simulink model "driver_model_vehicledynamics"  (R2023b)
settings: Solver=VariableStepAuto  StartTime=0  StopTime=100  FixedStep=0.001  RelTol=1e-3  AbsTol=1e-6
InitFcn:
  | R2D = 180/pi;
libraries: slpidlib x2, Solver_SF x1
settings Model: Creator=jhu  LastModifiedBy=rkddp
settings SolverCC: AutoScaleAbsTol=off  AlgebraicLoopSolver=TrustRegion
settings DataIOCC: SaveFormat=Array  SignalLoggingSaveFormat=ModelDataLogs  ReturnWorkspaceOutputs=off  SignalLoggingName=sigsOut
settings OptimizationCC: BlockReduction=off  BooleanDataType=off  ExpressionDepthLimit=2147483647  InitFltsAndDblsToZero=on  LifeSpan=inf
settings DebuggingCC: SaveWithParameterizedLinksMsg=none  UnderspecifiedInitializationDetection=Classic  MergeDetectMultiDrivingBlocksExec=none  SignalResolutionControl=TryResolveAllWithWarning  MultiTaskDSMMsg=warning  MultiTaskCondExecSysMsg=none  FcnCallInpInsideContextMsg=warning  UnconnectedInputMsg=warning  UnconnectedOutputMsg=warning  UnconnectedLineMsg=warning  StateNameClashWarn=warning  SFUnexpectedBacktrackingDiag=warning  SFNoUnconditionalDefaultTransitionDiag=warning  ArithmeticOperatorsInVariantConditions=warning
settings HardwareCC: ProdBitPerPointer=32  ProdBitPerSizeT=32  ProdBitPerPtrDiffT=32  ProdLargestAtomicFloat=None  ProdIntDivRoundTo=Undefined  ProdEndianess=Unspecified  ProdWordSize=32  ProdHWDeviceType=32-bit Generic  TargetHWDeviceType=32-bit Generic  TargetUnknown=on  ProdEqTarget=off
settings ModelReferenceCC: PropagateSignalLabelsOutOfModel=off
settings SFSimCC: SimUseLocalCustomCode=off  CustomCodeUndefinedFunction=UseInterfaceOnly
settings RTWCC: TemplateMakefile=grt_vc.tmf  RTWUseLocalCustomCode=off
settings CodeAppCC: StateflowObjectComments=on
settings GRTTargetCC: TargetFcnLib=ansi_tfl_tmw.mat  TargetLangStandard=C89/C90 (ANSI)  CombineOutputUpdateFcns=off  GRTInterface=on
settings ConfigComp: CovMetricSettings=dw  CovSaveCumulativeToWorkspaceVar=on  CovSaveSingleToWorkspaceVar=on  CovExternalEMLEnable=off

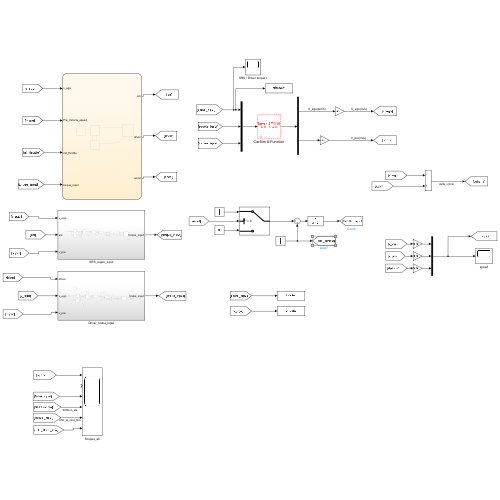
[thumbnail: Simulink's stored preview of the top-level diagram]
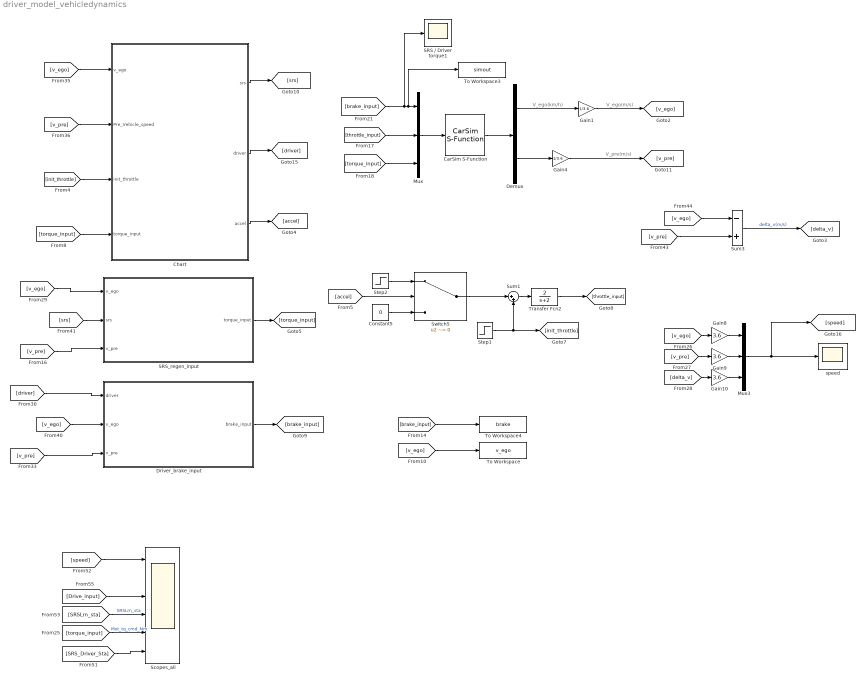
== system driver_model_vehicledynamics ==
  note: V_ego(m/s)
  note: V_pre(m/s)
  note: V_ego(km/h)
  CarSim S-Function : Solver_SF/CarSim S-Function  Priority=1  SIMFILE=simfile.sim  Run_RTs=off  vs_state_ind=Run  StopMode_ind=Vehicle Model
  Chart : Stateflow chart  TreatAsAtomicUnit=on
  Constant5 : Constant  Value=0
  Demux : Demux  Outputs=2
  Driver_brake_input : Subsystem
  Gain1 : Gain  Gain=1/3.6
  Gain10 : Gain  Gain=3.6
  Gain4 : Gain  Gain=1/3.6
  Gain8 : Gain  Gain=3.6
  Gain9 : Gain  Gain=3.6
  Mux : Mux  Inputs=3
  Mux3 : Mux  Inputs=3
  SRS / Driver torque1 : Scope
  SRS_regen_input : Subsystem
  Scopes_all : Scope  NumInputPorts=6
  Step1 : Step  Time=25  Before=0.2  After=0  SampleTime=0
  Step2 : Step  Time=30  After=0.2  SampleTime=0
  Sum1 : Sum  Inputs=|++
  Sum3 : Sum  Inputs=-+
  Switch5 : Switch  Criteria=u2 ~= 0  SaturateOnIntegerOverflow=off  InputSameDT=off
  To Workspace : ToWorkspace  VariableName=v_ego  SaveFormat=Timeseries  SampleTime=-1
  To Workspace3 : ToWorkspace  VariableName=simout  SaveFormat=Timeseries  SampleTime=-1
  To Workspace4 : ToWorkspace  VariableName=brake  SaveFormat=Timeseries  SampleTime=-1
  Transfer Fcn2 : TransferFcn  Numerator=[2]  Denominator=[1 2]
  speed : Scope
  wires:
  Gain1/1 -> [v_ego]
  [brake_input] -> To Workspace4/1
  [v_ego] -> To Workspace/1
  Step1/1 -> Sum1/2, [init_throttle]
  [throttle_input] -> Mux/2
  [torque_input] -> Mux/3
  [brake_input] -> SRS / Driver torque1/1, To Workspace3/1, Mux/1
  Mux/1 -> CarSim S-Function/1
  [v_ego] -> Gain8/1
  [v_pre] -> Gain9/1
  [delta_v] -> Gain10/1
  [torque_input] -> Scopes_all/5  "Mot_tq_cmd_Nm"
  [v_ego] -> Chart/1(v_ego)
  [v_pre] -> Chart/2(Pre_Vehicle_speed)
  Chart/1(srs) -> [srs]
  Chart/2(driver) -> [driver]
  [init_throttle] -> Chart/3(init_throttle)
  Chart/3(accel) -> [accel]
  [accel] -> Switch5/2
  Constant5/1 -> Switch5/3
  Step2/1 -> Switch5/1
  Switch5/1 -> Sum1/1
  Sum1/1 -> Transfer Fcn2/1
  Mux3/1 -> [speed], speed/1
  [torque_input] -> Chart/4(torque_input)
  [v_ego] -> Driver_brake_input/2(v_ego)
  Driver_brake_input/1(brake_input) -> [brake_input]
  [v_ego] -> SRS_regen_input/1(v_ego)
  [driver] -> Driver_brake_input/1(driver)
  [srs] -> SRS_regen_input/2(srs)
  SRS_regen_input/1(torque_input) -> [torque_input]
  [v_pre] -> SRS_regen_input/3(v_pre)
  [v_pre] -> Driver_brake_input/3(v_pre)
  Transfer Fcn2/1 -> [throttle_input]
  Demux/1 -> Gain1/1
  Gain4/1 -> [v_pre]
  Demux/2 -> Gain4/1
  CarSim S-Function/1 -> Demux/1
  Gain8/1 -> Mux3/1
  Gain9/1 -> Mux3/2
  Gain10/1 -> Mux3/3
  [SRS_Driver_Sta] -> Scopes_all/6
  [SRSLrn_sta] -> Scopes_all/4  "SRSLrn_sta"
  [speed] -> Scopes_all/1
  [Drive_input] -> Scopes_all/3
  [v_ego] -> Sum3/1
  [v_pre] -> Sum3/2
  Sum3/1 -> [delta_v]  "delta_v(m/s)"

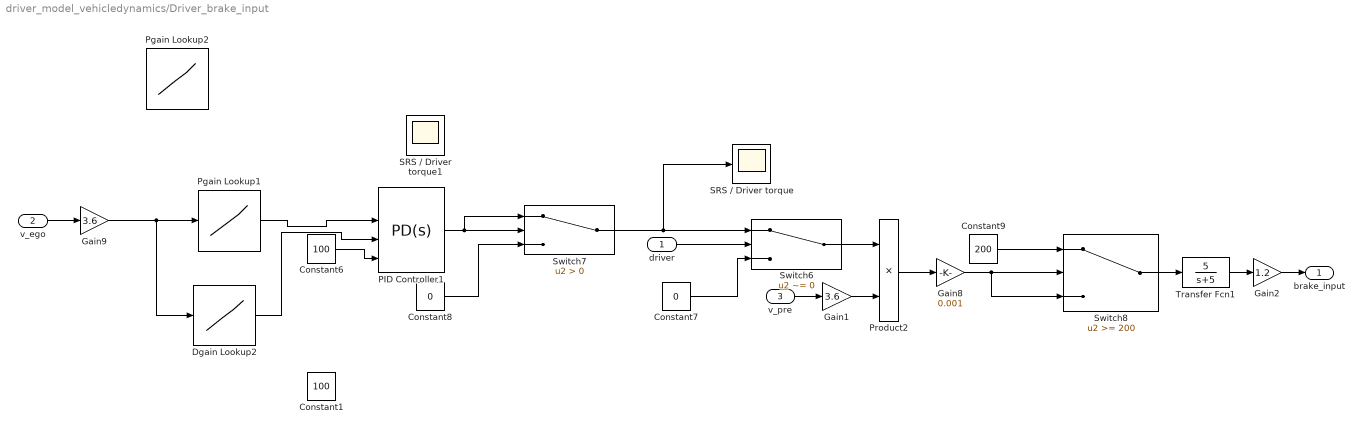
== system driver_model_vehicledynamics/Driver_brake_input ==
  driver : Inport
  v_ego : Inport  Port=2
  v_pre : Inport  Port=3
  Constant1 : Constant  Value=100
  Constant6 : Constant  Value=100
  Constant7 : Constant  Value=0
  Constant8 : Constant  Value=0
  Constant9 : Constant  Value=200
  Dgain Lookup2 : Lookup_n-D  NumberOfTableDimensions=1  BreakpointsForDimension1=[0 10 20 30 40 50 60 70 80 90]  Table=[100 100 100 100 100 100 100 300 300 300]  InternalRulePriority=Speed  RndMeth=Simplest
  Gain1 : Gain  Gain=3.6
  Gain2 : Gain  Gain=1.2
  Gain8 : Gain  Gain=0.001
  Gain9 : Gain  Gain=3.6
  PID Controller1 : slpidlib/PID Controller  Controller=PD  Form=Parallel  TimeDomain=Continuous-time  UseExternalTs=off  SampleTime=-1  IntegratorMethod=Forward Euler  FilterMethod=Forward Euler  ControllerParametersSource=external  P=1  I=1  UseKiTs=off  D=0  N=100  UseFilter=on  TunerSelectOption=Transfer Function Based (PID Tuner App)  InitialConditionSource=internal  InitialConditionForIntegrator=0  InitialConditionForFilter=0  DifferentiatorICPrevScaledInput=0  ExternalReset=none  TrackingMode=off  Kt=1  LimitOutput=off  SatLimitsSource=internal  UpperSaturationLimit=inf  LowerSaturationLimit=-inf  LinearizeAsGain=on  AntiWindupMode=none  Kb=1  LimitIntegrator=off  UpperIntegratorSaturationLimit=inf  LowerIntegratorSaturationLimit=-inf  POutMin=[]  POutMax=[]  IOutMin=[]  IOutMax=[]  DOutMin=[]  DOutMax=[]  NOutMin=[]  NOutMax=[]  SumOutMin=[]  SumOutMax=[]  SaturationOutMin=[]  SaturationOutMax=[]  PParamMin=[]  PParamMax=[]  IParamMin=[]  IParamMax=[]  DParamMin=[]  DParamMax=[]  NParamMin=[]  NParamMax=[]  KbParamMin=[]  KbParamMax=[]  KtParamMin=[]  KtParamMax=[]  KbOutMin=[]  KbOutMax=[]  KtOutMin=[]  KtOutMax=[]  IntegratorOutMin=[]  IntegratorOutMax=[]  FilterOutMin=[]  FilterOutMax=[]  SumI1OutMin=[]  SumI1OutMax=[]  SumI2OutMin=[]  SumI2OutMax=[]  SumI3OutMin=[]  SumI3OutMax=[]  SumI4OutMin=[]  SumI4OutMax=[]  SumDOutMin=[]  SumDOutMax=[]  DifferentiatorOutMin=[]  DifferentiatorOutMax=[]  FilterDiffOutCoefMin=[]  FilterDiffOutCoefMax=[]  ReciprocalOutMin=[]  ReciprocalOutMax=[]  SumDenOutMin=[]  SumDenOutMax=[]  SumNumOutMin=[]  SumNumOutMax=[]  DivideOutMin=[]  DivideOutMax=[]  UdiffTsProdOutMin=[]  UdiffTsProdOutMax=[]  NTsProdOutMin=[]  NTsProdOutMax=[]  UintegralTsProdOutMin=[]  UintegralTsProdOutMax=[]  UngainTsProdOutMin=[]  UngainTsProdOutMax=[]  ClampingZeroOutDataTypeStr=Inherit: Inherit via back propagation  ClampingZeroOutMin=[]  ClampingZeroOutMax=[]  FilterDenConstantOutDataTypeStr=Inherit: Inherit via back propagation  FilterDenConstantOutMin=[]  FilterDenConstantOutMax=[]  PCopyOutDataTypeStr=Inherit: Inherit via back propagation  PCopyOutMin=[]  PCopyOutMax=[]  NCopyOutDataTypeStr=Inherit: Inherit via back propagation  NCopyOutMin=[]  NCopyOutMax=[]  IntegratorContinuousStateAttributes=''  IntegratorStateMustResolveToSignalObject=off  IntegratorRTWStateStorageClass=Auto  FilterContinuousStateAttributes=''  FilterStateMustResolveToSignalObject=off  FilterRTWStateStorageClass=Auto  ParallelPVariant=ExternalParameters  IdealPVariant=Disabled  IVariant=Disabled  DVariant=ExternalParameters  IntegratorVariant=Disabled  SatVariant=Disabled  AWVariant=Disabled  PCopyVariant=Disabled  TRVariant=Disabled  FdbkBlocksVariant=Forward  IdealPFdbkVariant=Disabled  SatFdbkVariant=Disabled  DerivativeFilterVariant=ContFilter  NVariant=ExternalParameters  NCopyVariant=Disabled  FilterICVariant=InternalICsFilter  IntegratorICVariant=Disabled  ExternalResetVariant=Disabled  TRSumVariant=Passthrough  SumFdbkVariant=Disabled  SumVariant=Sum_PD  TsampFilterVariant=InternalTs  TsampNgainVariant=Passthrough  TsampIntegralVariant=Disabled_SignalSpec  ExternalSaturationOutDataTypeStr=Inherit: Same as second input
  Pgain Lookup1 : Lookup_n-D  NumberOfTableDimensions=1  BreakpointsForDimension1=[0 10 20 30 40 50 60 70 80 90]  Table=[300 300 270 250 250 250 270 300 300 300]  InternalRulePriority=Speed  RndMeth=Simplest
  Pgain Lookup2 : Lookup_n-D  NumberOfTableDimensions=1  BreakpointsForDimension1=[0 10 20 30 40 50 60 70 80 90]  Table=[300 300 100 100 300 300 100 500 300 300]  InternalRulePriority=Speed  RndMeth=Simplest
  Product2 : Product  SaturateOnIntegerOverflow=on  OutDataTypeStr=Inherit: Same as first input
  SRS / Driver torque : Scope
  SRS / Driver torque1 : Scope
  Switch6 : Switch  Criteria=u2 ~= 0  SaturateOnIntegerOverflow=off  InputSameDT=off
  Switch7 : Switch  Criteria=u2 > Threshold  SaturateOnIntegerOverflow=off  InputSameDT=off
  Switch8 : Switch  Threshold=200  SaturateOnIntegerOverflow=off  InputSameDT=off
  Transfer Fcn1 : TransferFcn  Numerator=[5]  Denominator=[1 5]
  brake_input : Outport
  wires:
  Constant6/1 -> PID Controller1/4
  PID Controller1/1 -> Switch7/2, Switch7/1
  Constant9/1 -> Switch8/1
  Product2/1 -> Gain8/1
  Constant7/1 -> Switch6/3
  Constant8/1 -> Switch7/3
  Switch7/1 -> SRS / Driver torque/1, Switch6/1
  v_ego/1 -> Gain9/1
  Switch6/1 -> Product2/1
  driver/1 -> Switch6/2
  v_pre/1 -> Gain1/1
  Gain1/1 -> Product2/2
  Gain9/1 -> Dgain Lookup2/1, Pgain Lookup1/1
  Dgain Lookup2/1 -> PID Controller1/3
  Pgain Lookup1/1 -> PID Controller1/2
  Gain8/1 -> Switch8/3, Switch8/2
  Switch8/1 -> Transfer Fcn1/1
  Transfer Fcn1/1 -> Gain2/1
  Gain2/1 -> brake_input/1

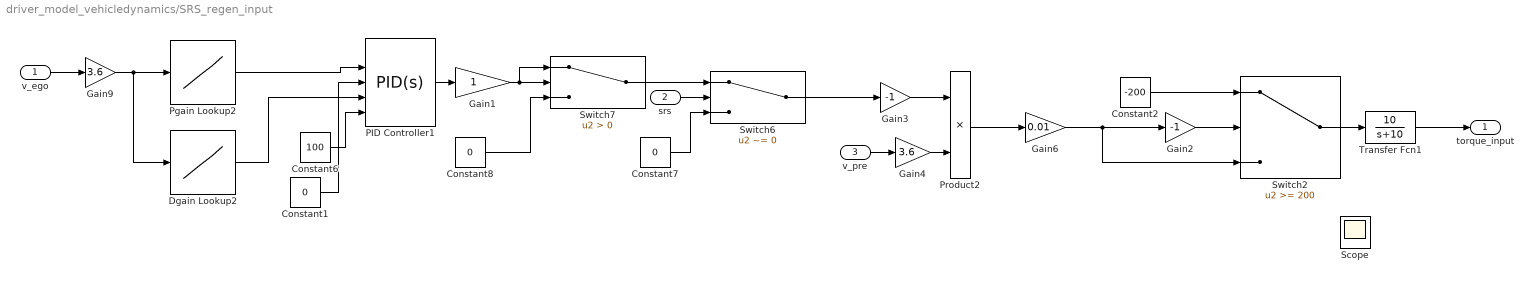
== system driver_model_vehicledynamics/SRS_regen_input ==
  v_ego : Inport
  srs : Inport  Port=2
  v_pre : Inport  Port=3
  Constant1 : Constant  Value=0
  Constant2 : Constant  Value=-200
  Constant6 : Constant  Value=100
  Constant7 : Constant  Value=0
  Constant8 : Constant  Value=0
  Dgain Lookup2 : Lookup_n-D  NumberOfTableDimensions=1  BreakpointsForDimension1=[0 10 20 30 40 50 60 70 80 90]  Table=[500 800 800 300 300 300 300 1000 1000 100]  InternalRulePriority=Speed  RndMeth=Simplest
  Gain1 : Gain
  Gain2 : Gain  Gain=-1
  Gain3 : Gain  Gain=-1
  Gain4 : Gain  Gain=3.6
  Gain6 : Gain  Gain=0.01
  Gain9 : Gain  Gain=3.6
  PID Controller1 : slpidlib/PID Controller  Controller=PID  Form=Parallel  TimeDomain=Continuous-time  UseExternalTs=off  SampleTime=-1  IntegratorMethod=Forward Euler  FilterMethod=Forward Euler  ControllerParametersSource=external  P=1  I=1  UseKiTs=off  D=0  N=100  UseFilter=on  TunerSelectOption=Transfer Function Based (PID Tuner App)  InitialConditionSource=internal  InitialConditionForIntegrator=0  InitialConditionForFilter=0  DifferentiatorICPrevScaledInput=0  ExternalReset=none  TrackingMode=off  Kt=1  LimitOutput=off  SatLimitsSource=internal  UpperSaturationLimit=inf  LowerSaturationLimit=-inf  LinearizeAsGain=on  AntiWindupMode=none  Kb=1  LimitIntegrator=off  UpperIntegratorSaturationLimit=inf  LowerIntegratorSaturationLimit=-inf  POutMin=[]  POutMax=[]  IOutMin=[]  IOutMax=[]  DOutMin=[]  DOutMax=[]  NOutMin=[]  NOutMax=[]  SumOutMin=[]  SumOutMax=[]  SaturationOutMin=[]  SaturationOutMax=[]  PParamMin=[]  PParamMax=[]  IParamMin=[]  IParamMax=[]  DParamMin=[]  DParamMax=[]  NParamMin=[]  NParamMax=[]  KbParamMin=[]  KbParamMax=[]  KtParamMin=[]  KtParamMax=[]  KbOutMin=[]  KbOutMax=[]  KtOutMin=[]  KtOutMax=[]  IntegratorOutMin=[]  IntegratorOutMax=[]  FilterOutMin=[]  FilterOutMax=[]  SumI1OutMin=[]  SumI1OutMax=[]  SumI2OutMin=[]  SumI2OutMax=[]  SumI3OutMin=[]  SumI3OutMax=[]  SumI4OutMin=[]  SumI4OutMax=[]  SumDOutMin=[]  SumDOutMax=[]  DifferentiatorOutMin=[]  DifferentiatorOutMax=[]  FilterDiffOutCoefMin=[]  FilterDiffOutCoefMax=[]  ReciprocalOutMin=[]  ReciprocalOutMax=[]  SumDenOutMin=[]  SumDenOutMax=[]  SumNumOutMin=[]  SumNumOutMax=[]  DivideOutMin=[]  DivideOutMax=[]  UdiffTsProdOutMin=[]  UdiffTsProdOutMax=[]  NTsProdOutMin=[]  NTsProdOutMax=[]  UintegralTsProdOutMin=[]  UintegralTsProdOutMax=[]  UngainTsProdOutMin=[]  UngainTsProdOutMax=[]  ClampingZeroOutDataTypeStr=Inherit: Inherit via back propagation  ClampingZeroOutMin=[]  ClampingZeroOutMax=[]  FilterDenConstantOutDataTypeStr=Inherit: Inherit via back propagation  FilterDenConstantOutMin=[]  FilterDenConstantOutMax=[]  PCopyOutDataTypeStr=Inherit: Inherit via back propagation  PCopyOutMin=[]  PCopyOutMax=[]  NCopyOutDataTypeStr=Inherit: Inherit via back propagation  NCopyOutMin=[]  NCopyOutMax=[]  IntegratorContinuousStateAttributes=''  IntegratorStateMustResolveToSignalObject=off  IntegratorRTWStateStorageClass=Auto  FilterContinuousStateAttributes=''  FilterStateMustResolveToSignalObject=off  FilterRTWStateStorageClass=Auto  ParallelPVariant=ExternalParameters  IdealPVariant=Disabled  IVariant=ExternalParameters  DVariant=ExternalParameters  IntegratorVariant=Continuous  SatVariant=Disabled  AWVariant=Passthrough  PCopyVariant=Disabled  TRVariant=Disabled  FdbkBlocksVariant=Forward  IdealPFdbkVariant=Disabled  SatFdbkVariant=Disabled  DerivativeFilterVariant=ContFilter  NVariant=ExternalParameters  NCopyVariant=Disabled  FilterICVariant=InternalICsFilter  IntegratorICVariant=InternalICs  ExternalResetVariant=Disabled  TRSumVariant=Passthrough  SumFdbkVariant=Disabled  SumVariant=Sum_PID  TsampFilterVariant=InternalTs  TsampNgainVariant=Passthrough  TsampIntegralVariant=Disabled_SignalSpec  ExternalSaturationOutDataTypeStr=Inherit: Same as second input
  Pgain Lookup2 : Lookup_n-D  NumberOfTableDimensions=1  BreakpointsForDimension1=[0 10 20 30 40 50 60 70 80 90]  Table=[800 800 800 300 300 500 500 800 800 200]  InternalRulePriority=Speed  RndMeth=Simplest
  Product2 : Product  SaturateOnIntegerOverflow=on  OutDataTypeStr=Inherit: Same as first input
  Scope : Scope
  Switch2 : Switch  Threshold=200  SaturateOnIntegerOverflow=off  InputSameDT=off
  Switch6 : Switch  Criteria=u2 ~= 0  SaturateOnIntegerOverflow=off  InputSameDT=off
  Switch7 : Switch  Criteria=u2 > Threshold  SaturateOnIntegerOverflow=off  InputSameDT=off
  Transfer Fcn1 : TransferFcn  Numerator=[10]  Denominator=[1 10]
  torque_input : Outport
  wires:
  Constant6/1 -> PID Controller1/5
  PID Controller1/1 -> Gain1/1
  Pgain Lookup2/1 -> PID Controller1/2
  Gain9/1 -> Dgain Lookup2/1, Pgain Lookup2/1
  v_pre/1 -> Gain4/1
  Constant7/1 -> Switch6/3
  Dgain Lookup2/1 -> PID Controller1/4
  srs/1 -> Switch6/2
  Constant8/1 -> Switch7/3
  Switch7/1 -> Switch6/1
  v_ego/1 -> Gain9/1
  Product2/1 -> Gain6/1
  Gain1/1 -> Switch7/2, Switch7/1
  Transfer Fcn1/1 -> torque_input/1
  Gain2/1 -> Switch2/2
  Constant2/1 -> Switch2/1
  Constant1/1 -> PID Controller1/3
  Gain3/1 -> Product2/1
  Switch6/1 -> Gain3/1
  Gain4/1 -> Product2/2
  Switch2/1 -> Transfer Fcn1/1
  Gain6/1 -> Switch2/3, Gain2/1

== stateflow chart driver_model_vehicledynamics/Chart ==
  state SRS_ON
    en:
    driver = 0;
    srs = 1;
    SRSCnt=1;
    SRSCheck =+1;
    du:
    SRSCnt=SRSCnt+1;
    ex:
    SRSCnt=0;
  state OFF
    en:
    driver = 0;
    srs =0;
    accel = 0;
  state INIT
    en:
    driver = 0;
    srs =0;
    accel = 0;
    SRSCheck = 0;
    DriverCheck = 0;
    DriverCnt=0;
  state Driver_ON
    en:
    driver = 1;
    srs = 0;
    DriverCnt=1;
    DriverCheck = DriverCheck +1;
    du:
    DriverCnt=DriverCnt+1;
    ex:
    DriverCnt=0;
  (default) -> INIT
  OFF -> SRS_ON [order 2] : [ DriverCheck == 0 && Pre_Vehicle_speed - v_ego < 0  && init_throttle ==0  ]
  INIT -> OFF
  OFF -> Driver_ON [order 1] : [SRSCheck ~=0  && Pre_Vehicle_speed - v_ego < 0  && init_throttle ==0 ]
  Driver_ON -> OFF : [(Pre_Vehicle_speed - v_ego >= 0)]
  SRS_ON -> Driver_ON : [(v_ego <1 && SRSCnt > 2000) || (Pre_Vehicle_speed - v_ego >= 0 && SRSCnt > 2000 ) || SRSCnt > 2000]
  data: srs output; driver output; accel output; v_ego input; Pre_Vehicle_speed input; init_throttle input; DriverCnt local; torque_input input; SRSCnt local; DriverCheck local; SRSCheck local
